simulink library "Hydraulic_Actuator_Lib"  (R2019b)
settings: Solver=ode45  StartTime=0.0  StopTime=10.0  RelTol=1e-3  EnableMultiTasking=on
undefined symbols (not defined in the file): WT_Params
libraries: fl_lib x15, sh_lib x9, nesl_utility x9, fl_ps_legacy_lib x4
Description:
  | Copyright 2009-2017 The MathWorks, Inc. MathWorks, Inc.
settings Model: Creator=smiller  LastModifiedBy=bhisma
settings DataIOCC: LimitDataPoints=on  SaveFormat=Array  SignalLoggingSaveFormat=ModelDataLogs  ReturnWorkspaceOutputs=off
settings OptimizationCC: ExpressionDepthLimit=2147483647  LifeSpan=inf
settings DebuggingCC: UnderspecifiedInitializationDetection=Classic  MergeDetectMultiDrivingBlocksExec=none  SolverPrmCheckMsg=warning  FcnCallInpInsideContextMsg=warning  AllowSymbolicDim=off  StateNameClashWarn=warning  SFUnexpectedBacktrackingDiag=warning  SFNoUnconditionalDefaultTransitionDiag=warning  SFExecutionAtInitializationDiag=none  ArithmeticOperatorsInVariantConditions=warning
settings HardwareCC: ProdBitPerPointer=32  ProdBitPerSizeT=32  ProdBitPerPtrDiffT=32  ProdLargestAtomicFloat=None  ProdIntDivRoundTo=Undefined  ProdEndianess=Unspecified  ProdWordSize=32  ProdHWDeviceType=32-bit Generic
settings ModelReferenceCC: PropagateSignalLabelsOutOfModel=off
settings SFSimCC: SimUseLocalCustomCode=off  CustomCodeUndefinedFunction=UseInterfaceOnly
settings RTWCC: RTWUseLocalCustomCode=off
settings CodeAppCC: StateflowObjectComments=on
settings GRTTargetCC: TargetLangStandard=C89/C90 (ANSI)  GeneratePreprocessorConditionals=Disable all  CombineOutputUpdateFcns=off  GRTInterface=on
settings ConfigComp: CovMetricSettings=dw  CovHtmlReporting=on  CovSaveCumulativeToWorkspaceVar=on  CovSaveSingleToWorkspaceVar=on  CovExternalEMLEnable=off  CovSFcnEnable=off

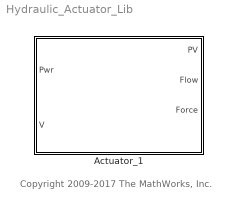
== system Hydraulic_Actuator_Lib ==
  note: Copyright 2009-2017 The MathWorks, Inc.
  Actuator_1 : Subsystem
      mask Display: image(imread('Pitch_Hydraulic_Actuator_IMAGE.jpg'));

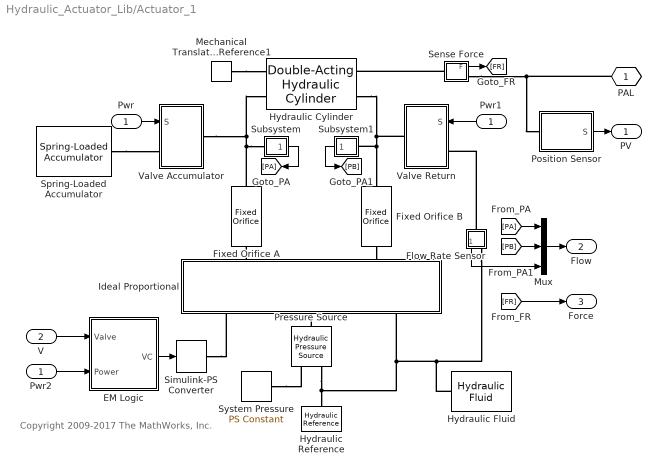
== system Hydraulic_Actuator_Lib/Actuator_1 ==
  note: Copyright 2009-2017 The MathWorks, Inc.
  Pwr : Inport
  V : Inport  Port=2
  EM Logic : Subsystem
  Fixed Orifice A : sh_lib/Orifices/Fixed Orifice  area=WT_Params.Pitch_Actuator.orifice_area m^2  C_d=0.7  lam_spec=2  B_lam=0.999  Re_cr=12  q_specify=off  q_priority=High  q=1 m^3/s  q_nominal_specify=off  q_nominal_unit=m^3/s  q_nominal_value=1  p_specify=off  p_priority=High  p=0 Pa  p_nominal_specify=off  p_nominal_unit=Pa  p_nominal_value=1
      settings: SourceProductName=Simscape Fluids  SourceProductBaseCode=SH  InternalSimscapePortConfiguration="{\"Bottom\":[],\"Left\":[{\"id\":\"A\",\"label\":\"A\",\"type\":\"foundation.hydraulic.hydraulic\"}],\"Right\":[{\"id\":\"B\",\"label\":\"B\",\"type\":\"foundation.hydraulic.hydraulic\"}],\"Top\":[]}"
  Fixed Orifice B : sh_lib/Orifices/Fixed Orifice  area=WT_Params.Pitch_Actuator.orifice_area m^2  C_d=0.7  lam_spec=2  B_lam=0.999  Re_cr=12  q_specify=off  q_priority=High  q=1 m^3/s  q_nominal_specify=off  q_nominal_unit=m^3/s  q_nominal_value=1  p_specify=off  p_priority=High  p=0 Pa  p_nominal_specify=off  p_nominal_unit=Pa  p_nominal_value=1
      settings: SourceProductName=Simscape Fluids  SourceProductBaseCode=SH  InternalSimscapePortConfiguration="{\"Bottom\":[],\"Left\":[{\"id\":\"A\",\"label\":\"A\",\"type\":\"foundation.hydraulic.hydraulic\"}],\"Right\":[{\"id\":\"B\",\"label\":\"B\",\"type\":\"foundation.hydraulic.hydraulic\"}],\"Top\":[]}"
  Flow Rate Sensor : Subsystem
      mask Display: disp('F')
  Hydraulic Reference : fl_lib/Hydraulic/Hydraulic Elements/Hydraulic Reference
      settings: SourceProductName=Simscape
  Hydraulic Cylinder : sh_lib/Hydraulic Cylinders/Double-Acting Hydraulic Cylinder  area_A=WT_Params.Pitch_Actuator.Cylinder.piston_area m^2  area_B=WT_Params.Pitch_Actuator.Cylinder.piston_area m^2  stroke=WT_Params.Pitch_Actuator.Cylinder.stroke m  init_pos=WT_Params.Pitch_Actuator.Cylinder.initial_disp_from_a m  dead_vol_A=1e-04 m^3  dead_vol_B=1e-04 m^3  init_pressure_A=0 Pa  init_pressure_B=0 Pa  k_sh=1.4  stiff=WT_Params.Pitch_Actuator.Cylinder.contact_stiffness N/m  D=WT_Params.Pitch_Actuator.Cylinder.contact_damping N/(m/s)  hardstop_model=3  transition=0.1 mm  or=2
      settings: SourceProductName=Simscape Fluids  SourceProductBaseCode=SH  InternalSimscapePortConfiguration="{\"Bottom\":[],\"Left\":[{\"id\":\"C\",\"label\":\"C\",\"type\":\"foundation.mechanical.translational.translational\"},{\"id\":\"A\",\"label\":\"A\",\"type\":\"foundation.hydraulic.hydraulic\"}],\"Right\":[{\"id\":\"R\",\"label\":\"R\",\"type\":\"foundation.mechanical.translational.translational\"},{\"id\":\"B\",\"label\":\"B\",\"type\":\"foundation.hydraulic.hydraulic\"}],\"Top\":[]}"
  Hydraulic Fluid : sh_lib/Hydraulic Utilities/Hydraulic Fluid  DataSource=1  SelFluid=1  SysTemp=60  TrapAir=0.005  ViscDerFactor=1  range_error=2
      settings: SourceProductName=Simscape Fluids
  Ideal Proportional : Subsystem
      mask Display:
      | plot([198.418507352471;198.418507352471], [5.66910021007061;25.5109509453177])
      | plot([189.914857037365;206.922157667577], [25.5109509453177;25.5109509453177])
      | plot([240.936758928001;240.936758928001], [5.66910021007061;25.5109509453177])
      | plot([232.433108612895;249.440409243107], [25.5109509453177;25.5109509453177])
      | plot([240.936758928001;240.936758928001], [76.5328528359532;56.6910021007061])
      | plot([232.433108612895;249.440409243107], [56.6910021007061;56.6910021007061])
      | plot([198.418507352471;198.418507352471], [76.5328528359532;56.6910021007061])
      | plot([189.914857037365;206.922157667577], [56.6910021007061;56.6910021007061])
      | plot([99.2092536762357;99.2092536762357], [76.5328528359532;5.66910021007061])
      | plot([141.727505251765;141.727505251765], [76.5328528359532;5.66910021007061])
      | plot([170.073006302118;170.073006302118], [76.5328528359532;5.66910021007061])
      | plot([269.282259978354;269.282259978354], [76.5328528359532;5.66910021007061])
      | patch([99.2092536762357;93.5401534661651;104.878353886306;99.2092536762357], [76.5328528359532;53.8564519956708;53.8564519956708;76.5328528359532],[0 0 0])
      | plot([99.2092536762357;93.5401534661651;104.878353886306;99.2092536762357], [76.5328528359532;53.8564519956708;53.8564519956708;76.5328528359532])
      | patch([141.727505251765;136.058405041695;147.396605461836;141.727505251765], [5.66910021007061;28.3455010503531;28.3455010503531;5.66910021007061],[0 0 0])
      | plot([141.727505251765;136.058405041695;147.396605461836;141.727505251765], [5.66910021007061;28.3455010503531;28.3455010503531;5.66910021007061])
      | plot([297.627761028707;340.146012604237], [5.66910021007061;76.5328528359532])
      | plot([297.627761028707;340.146012604237], [76.5328528359532;5.66910021007061])
      | plot([70.8637526258826;368.49151365459;368.49151365459;70.8637526258826;70.8637526258826], [76.5328528359532;76.5328528359532;5.66910021007061;5.66910021007061;76.5328528359532])
      | patch([297.627761028707;303.296861238778;311.800511553884;297.627761028707], [5.66910021007061;25.5109509453177;19.8418507352471;5.66910021007061],[0 0 0])
      | plot([297.627761028707;303.296861238778;311.800511553884;297.627761028707], [5.66910021007061;25.5109509453177;19.8418507352471;5.66910021007061])
      | patch([297.627761028707;303.296861238778;311.800511553884;297.627761028707], [76.5328528359532;56.6910021007061;62.3601023107767;76.5328528359532],[0 0 0])
      | plot([297.627761028707;303.296861238778;311.800511553884;297.627761028707], [76.5328528359532;56.6910021007061;62.3601023107767;76.5328528359532])
      | plot([62.3601023107767;374.16061386466], [82.2019530460238;82.2019530460238])
      | plot([65.194652415812;376.995163969696], [0;0])
      | plot([70.8637526258826;0;0;70.8637526258826;70.8637526258826], [53.8564519956708;53.8564519956708;25.5109509453177;25.5109509453177;53.8564519956708]-25.5109509453177+5.66910021007061)
      | plot([70.8637526258826;0;0;70.8637526258826;70.8637526258826]+368.49151365459, [53.8564519956708;53.8564519956708;25.5109509453177;25.5109509453177;53.8564519956708]-25.5109509453177+5.66910021007061)
      | plot([15 25], [5.66910021007061 35])
      | plot([25 15]+405, [5.66910021007061 35])
      | plot([42.5 40]+5,[70 58]);
      | plot([45 50]+2.5,[70 45]);
      | plot([45 50]+7.5,[45 70]);
      | plot([45 50]+12.5,[70 45]);
      | plot([45 50]+17.5,[45 70]);
      | plot([40 42.5]+27.5,[70 58]);
      | plot([42.5 40]+5+324,[70 58]);
      | plot([45 50]+2.5+324,[70 45]);
      | plot([45 50]+7.5+324,[45 70]);
      | plot([45 50]+12.5+324,[70 45]);
      | plot([45 50]+17.5+324,[45 70]);
      | plot([40 42.5]+27.5+324,[70 58]);
      | ;color('red');
      | port_label('LConn', 1,'A')
      | port_label('LConn', 2,'B')
      | port_label('RConn', 1,'S')
      | port_label('RConn', 2,'P')
      | port_label('RConn', 3,'T')
  Mechanical Translational Reference1 : fl_lib/Mechanical/Translational Elements/Mechanical Translational Reference  Tag=Factory Generic
  Mux : Mux  Inputs=3
  Position Sensor : Subsystem
      mask Display:
      | plot([25.5109509453177;56.6910021007061;70.8637526258826;96.3747035712004;127.554754726589;155.900255776942;184.245756827295;212.591257877648;235.26765871793;252.274959348142;283.455010503531], [155.900255776942;155.900255776942;110.547454096377;198.418507352471;113.382004201412;198.418507352471;116.216554306448;198.418507352471;113.382004201412;155.900255776942;155.900255776942])
      | plot([155.900255776942;155.900255776942], [266.447709873319;198.418507352471])
      | patch([155.900255776942;170.073006302118;141.727505251765;155.900255776942], [198.418507352471;226.764008402824;226.764008402824;198.418507352471], [0;0;0])
      | plot([155.900255776942;170.073006302118;141.727505251765;155.900255776942], [198.418507352471;226.764008402824;226.764008402824;198.418507352471])
      | ;
      | color('red');
      | port_label('LConn', 1,'R')
      | port_label('output', 1,'P')
  Pressure Source : fl_lib/Hydraulic/Hydraulic Sources/Hydraulic Pressure Source
      settings: SourceProductName=Simscape  SourceProductBaseCode=SS  InternalSimscapePortConfiguration="{\"Bottom\":[],\"Left\":[{\"id\":\"P\",\"label\":\"P\",\"type\":\"foundation.hydraulic.hydraulic\"}],\"Right\":[{\"id\":\"S\",\"label\":\"S\",\"type\":\"input\"},{\"id\":\"T\",\"label\":\"T\",\"type\":\"foundation.hydraulic.hydraulic\"}],\"Top\":[]}"
  Pwr1 : InportShadow
  Pwr2 : InportShadow
  Sense Force : Subsystem
      mask Display: disp('F');
  Simulink-PS Converter : nesl_utility/Simulink-PS Converter  PhysicalDomain=network_engine_domain  SubClassName=ps_input  LeftPortType=input  RightPortType=output  PseudoPeriodic=off  Frequencies=[]  NoiseDistribution=none  NoiseParameters=[]  Unit=1  AffineConversion=off  FilteringAndDerivatives=zero  SimscapeFilterOrder=1  InputFilterTimeConstant=.001  UdotUserProvided=0
  Spring-Loaded Accumulator : sh_lib/Accumulators/Spring-Loaded Accumulator  capacity=WT_Params.Pitch_Actuator.Accumulator.capacity m^3  pr_preload=WT_Params.Pitch_Actuator.Accumulator.preload_pressure Pa  pr_max=WT_Params.Pitch_Actuator.Accumulator.maximum_pressure Pa  stiff_coeff=0 Pa/m^3  penetr_coeff=1e15 s*Pa/m^6  flow_rate_specify=off  flow_rate_priority=None  flow_rate=0.005 m^3/s  flow_rate_nominal_specify=off  flow_rate_nominal_unit=m^3/s  flow_rate_nominal_value=1  fluid_volume_specify=on  fluid_volume_priority=High  fluid_volume=WT_Params.Pitch_Actuator.Accumulator.initial_volume m^3  fluid_volume_nominal_specify=off  fluid_volume_nominal_unit=m^3  fluid_volume_nominal_value=1  fluid_pressure_specify=off  fluid_pressure_priority=None  fluid_pressure=1.01325e+5 Pa  fluid_pressure_nominal_specify=off  fluid_pressure_nominal_unit=Pa  fluid_pressure_nominal_value=1
      settings: SourceProductName=Simscape Fluids  SourceProductBaseCode=SH  InternalSimscapePortConfiguration="{\"Bottom\":[],\"Left\":[],\"Right\":[{\"id\":\"A\",\"label\":\"A\",\"type\":\"foundation.hydraulic.hydraulic\"}],\"Top\":[]}"
  Subsystem : Subsystem
      mask Display: disp('P')
  Subsystem1 : Subsystem
      mask Display: disp('P')
  System Pressure : fl_lib/Physical Signals/Sources/PS Constant  constant=WT_Params.Pitch_Actuator.hydraulic_pressure
  Valve Accumulator : Subsystem
      mask Display:
      | plot([73.6983027309179;124.720204621553], [181.41120672226;181.41120672226])
      | plot([76.2808928266168;277.78591029346], [385.498814284801;385.498814284801])
      | plot([77.0997628569603;276.967040263116], [283.455010503531;283.455010503531])
      | plot([73.6983027309179;276.967040263116;276.967040263116;73.6983027309179;73.6983027309179], [487.542618066072;487.542618066072;79.3674029409885;79.3674029409885;487.542618066072])
      | plot([277.78591029346;226.764008402824], [181.41120672226;181.285226717591])
      | plot([226.764008402824;226.764008402824], [205.28441760689;157.286035828292])
      | patch([206.35524764657;206.35524764657;280.368500389159;206.35524764657], [400.805384851992;370.192243717611;385.498814284801;400.805384851992], [0;0;0])
      | plot([206.35524764657;206.35524764657;280.368500389159;206.35524764657], [400.805384851992;370.192243717611;385.498814284801;400.805384851992])
      | plot([124.720204621553;124.720204621553], [204.906477592885;156.971085816622])
      | plot([0;351.484213024378;351.484213024378;0;0], [566.910021007061;566.910021007061;0;0;566.910021007061])
      | ;
      | color('red');
      | port_label('input', 1,'S');
      | port_label('lconn', 1,'A');
      | port_label('rconn', 1,'B');
  Valve Return : Subsystem
      mask Display:
      | plot([73.6983027309179;124.720204621553], [181.41120672226;181.41120672226])
      | plot([76.2808928266168;277.78591029346], [385.498814284801;385.498814284801])
      | plot([77.0997628569603;276.967040263116], [283.455010503531;283.455010503531])
      | plot([73.6983027309179;276.967040263116;276.967040263116;73.6983027309179;73.6983027309179], [487.542618066072;487.542618066072;79.3674029409885;79.3674029409885;487.542618066072])
      | plot([277.78591029346;226.764008402824], [181.41120672226;181.285226717591])
      | plot([226.764008402824;226.764008402824], [205.28441760689;157.286035828292])
      | patch([206.35524764657;206.35524764657;280.368500389159;206.35524764657], [400.805384851992;370.192243717611;385.498814284801;400.805384851992], [0;0;0])
      | plot([206.35524764657;206.35524764657;280.368500389159;206.35524764657], [400.805384851992;370.192243717611;385.498814284801;400.805384851992])
      | plot([124.720204621553;124.720204621553], [204.906477592885;156.971085816622])
      | plot([0;351.484213024378;351.484213024378;0;0], [566.910021007061;566.910021007061;0;0;566.910021007061])
      | ;
      | color('red');
      | port_label('input', 1,'S');
      | port_label('lconn', 1,'A');
      | port_label('rconn', 1,'B');
  PAL : PMIOPort  Tag=PMCPort  Side=Right
  PV : Outport
  Flow : Outport  Port=2
  Force : Outport  Port=3
  wires:
  Pwr2/1 -> EM Logic/2(Power)
  EM Logic/1(VC) -> Simulink-PS Converter/1
  [PB] -> Mux/2
  [PA] -> Mux/1
  Flow Rate Sensor/1(Flow) -> Mux/3
  Subsystem1/1(P) -> [PB]
  Subsystem/1(P) -> [PA]
  V/1 -> EM Logic/1(Valve)
  Pwr1/1 -> Valve Return/1(S)
  Pwr/1 -> Valve Accumulator/1(S)
  Position Sensor/1(S) -> PV/1
  Mux/1 -> Flow/1
  Sense Force/1(F) -> [FR]
  [FR] -> Force/1
  connections:
  Flow Rate Sensor/LConn1 -- Valve Return/LConn1
  Sense Force/RConn1 -- PAL/RConn1 -- Position Sensor/LConn1
  Spring-Loaded Accumulator/RConn1 -- Valve Accumulator/LConn1
  Mechanical Translational Reference1/LConn1 -- Hydraulic Cylinder/LConn1
  Subsystem/LConn1 -- Fixed Orifice A/RConn1 -- Valve Accumulator/RConn1 -- Hydraulic Cylinder/LConn2
  Subsystem1/LConn1 -- Valve Return/RConn1 -- Hydraulic Cylinder/RConn2 -- Fixed Orifice B/RConn1
  Ideal Proportional/LConn1 -- Fixed Orifice A/LConn1
  Fixed Orifice B/LConn1 -- Ideal Proportional/LConn2
  Ideal Proportional/RConn3 -- Hydraulic Reference/LConn1 -- Pressure Source/RConn2 -- Hydraulic Fluid/RConn1 -- Flow Rate Sensor/RConn1
  Simulink-PS Converter/RConn1 -- Ideal Proportional/RConn1
  Pressure Source/LConn1 -- Ideal Proportional/RConn2
  System Pressure/RConn1 -- Pressure Source/RConn1
  Sense Force/LConn1 -- Hydraulic Cylinder/RConn1

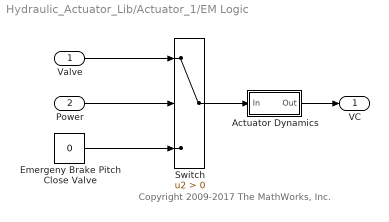
== system Hydraulic_Actuator_Lib/Actuator_1/EM Logic ==
  note: Copyright 2009-2017 The MathWorks, Inc.
  Valve : Inport
  Power : Inport  Port=2
  Actuator Dynamics : Subsystem  mask(First-order lag supporting vector signals){b=WT_Params.Pitch_Actuator.hydraulic_actuator_time_constant, x_initial=0}
      mask prompts: b "Filter time constant"; x_initial "Initial output"
      mask help: Models a lag of the form 1/(b*s+1) where s is the Laplace operator.
  Emergeny Brake Pitch Close Valve : Constant  Value=0
  Switch : Switch  Criteria=u2 > Threshold
  VC : Outport
  wires:
  Switch/1 -> Actuator Dynamics/1(In)
  Emergeny Brake Pitch Close Valve/1 -> Switch/3
  Power/1 -> Switch/2
  Valve/1 -> Switch/1
  Actuator Dynamics/1(Out) -> VC/1

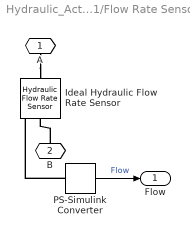
== system Hydraulic_Actuator_Lib/Actuator_1/Flow Rate Sensor ==
  Ideal Hydraulic Flow Rate Sensor : fl_lib/Hydraulic/Hydraulic Sensors/Hydraulic Flow Rate Sensor
      settings: SourceProductName=Simscape
  PS-Simulink Converter : nesl_utility/PS-Simulink Converter  PhysicalDomain=network_engine_domain  SubClassName=ps_output  LeftPortType=input  RightPortType=output  PseudoPeriodic=off  Frequencies=[]  Unit=1  AffineConversion=off
  A : PMIOPort  Side=Left
  B : PMIOPort  Port=2  Side=Right
  Flow : Outport
  wires:
  PS-Simulink Converter/1 -> Flow/1  "Flow"
  connections:
  B/RConn1 -- Ideal Hydraulic Flow Rate Sensor/RConn2
  A/RConn1 -- Ideal Hydraulic Flow Rate Sensor/LConn1
  PS-Simulink Converter/LConn1 -- Ideal Hydraulic Flow Rate Sensor/RConn1

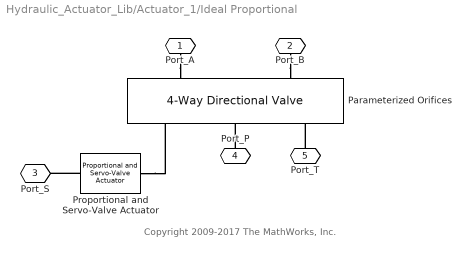
== system Hydraulic_Actuator_Lib/Actuator_1/Ideal Proportional ==
  note: Copyright 2009-2017 The MathWorks, Inc.
  Parameterized Orifices : sh_lib/Valves/Directional Valves/4-Way Directional Valve  area_spec=1  x_0_P_A=WT_Params.Pitch_Actuator.Valve.initial_opening_pa m  x_0_P_B=WT_Params.Pitch_Actuator.Valve.initial_opening_pb m  x_0_A_T=WT_Params.Pitch_Actuator.Valve.initial_opening_at m  x_0_B_T=WT_Params.Pitch_Actuator.Valve.initial_opening_bt m  mdl_type_identical=1  mdl_type_different=1  opening_max=WT_Params.Pitch_Actuator.Valve.max_opening m  area_max=WT_Params.Pitch_Actuator.Valve.max_area m^2  opening_max_P_A=0.005 m  area_max_P_A=0.5e-4 m^2  opening_max_P_B=0.005 m  area_max_P_B=0.5e-4 m^2  opening_max_A_T=0.005 m  area_max_A_T=0.5e-4 m^2  opening_max_B_T=0.005 m  area_max_B_T=0.5e-4 m^2  opening_area_tab="[  -0.002 0 0.002 0.005 0.015 ] m"  area_tab="[  1e-09 2.0352e-07 4.0736e-05 0.00011438 0.00034356 ] m^2"  opening_flow_rate_tab="[  -0.002 0 0.002 0.005 0.015 ] m"  pressure_tab="[  -1e+07 -5e+06 -2e+06 2e+06 5e+06 1e+07 ] Pa"  flow_rate_tab="[  -1e-07 -7.0711e-08 -4.4721e-08 4.4721e-08 7.0711e-08 1e-07 ; -2.0352e-05 -1.4391e-05 -9.1017e-06 9.1017e-06 1.4391e-05 2.0352e-05 ; -0.0040736 -0.0028805 -0.0018218 0.0018218 0.0028805 0.0040736 ; -0.011438 -0.0080879 -0.0051152 0.0051152 0.0080879 0.011438 ; -0.034356 -0.024293 -0.015364 0.015364 0.024293 0.034356 ; ] m^3/s"  opening_area_tab_P_A=[-0.002, 0.0, 0.002, 0.005, 0.015] m  area_tab_P_A=[1.0e-9, 2.0352e-7, 4.0736e-5, 0.00011438, 0.00034356] m^2  opening_flow_rate_tab_P_A=[-0.002, 0.0, 0.002, 0.005, 0.015] m  pressure_tab_P_A=[-10000000.0, -5000000.0, -2000000.0, 2000000.0, 5000000.0, 10000000.0] Pa  flow_rate_tab_P_A=[-1.0e-7, -7.0711e-8, -4.4721e-8, 4.4721e-8, 7.0711e-8, 1.0e-7; -2.0352e-5, -1.4391e-5, -9.1017e-6, 9.1017e-6, 1.4391e-5, 2.0352e-5; -0.0040736, -0.0028805, -0.0018218, 0.0018218, 0.0028805, 0.0040736; -0.011438, -0.0080879, -0.0051152, 0.0051152, 0.0080879, 0.011438; -0.034356, -0.024293, -0.015364, 0.015364, 0.024293, 0.034356] m^3/s  opening_area_tab_P_B=[-0.002, 0.0, 0.002, 0.005, 0.015] m  area_tab_P_B=[1.0e-9, 2.0352e-7, 4.0736e-5, 0.00011438, 0.00034356] m^2  opening_flow_rate_tab_P_B=[-0.002, 0.0, 0.002, 0.005, 0.015] m  pressure_tab_P_B=[-10000000.0, -5000000.0, -2000000.0, 2000000.0, 5000000.0, 10000000.0] Pa  flow_rate_tab_P_B=[-1.0e-7, -7.0711e-8, -4.4721e-8, 4.4721e-8, 7.0711e-8, 1.0e-7; -2.0352e-5, -1.4391e-5, -9.1017e-6, 9.1017e-6, 1.4391e-5, 2.0352e-5; -0.0040736, -0.0028805, -0.0018218, 0.0018218, 0.0028805, 0.0040736; -0.011438, -0.0080879, -0.0051152, 0.0051152, 0.0080879, 0.011438; -0.034356, -0.024293, -0.015364, 0.015364, 0.024293, 0.034356] m^3/s  opening_area_tab_A_T=[-0.002, 0.0, 0.002, 0.005, 0.015] m  area_tab_A_T=[1.0e-9, 2.0352e-7, 4.0736e-5, 0.00011438, 0.00034356] m^2  opening_flow_rate_tab_A_T=[-0.002, 0.0, 0.002, 0.005, 0.015] m  pressure_tab_A_T=[-10000000.0, -5000000.0, -2000000.0, 2000000.0, 5000000.0, 10000000.0] Pa  flow_rate_tab_A_T=[-1.0e-7, -7.0711e-8, -4.4721e-8, 4.4721e-8, 7.0711e-8, 1.0e-7; -2.0352e-5, -1.4391e-5, -9.1017e-6, 9.1017e-6, 1.4391e-5, 2.0352e-5; -0.0040736, -0.0028805, -0.0018218, 0.0018218, 0.0028805, 0.0040736; -0.011438, -0.0080879, -0.0051152, 0.0051152, 0.0080879, 0.011438; -0.034356, -0.024293, -0.015364, 0.015364, 0.024293, 0.034356] m^3/s  opening_area_tab_B_T=[-0.002, 0.0, 0.002, 0.005, 0.015] m  area_tab_B_T=[1.0e-9, 2.0352e-7, 4.0736e-5, 0.00011438, 0.00034356] m^2  opening_flow_rate_tab_B_T=[-0.002, 0.0, 0.002, 0.005, 0.015] m  pressure_tab_B_T=[-10000000.0, -5000000.0, -2000000.0, 2000000.0, 5000000.0, 10000000.0] Pa  flow_rate_tab_B_T=[-1.0e-7, -7.0711e-8, -4.4721e-8, 4.4721e-8, 7.0711e-8, 1.0e-7; -2.0352e-5, -1.4391e-5, -9.1017e-6, 9.1017e-6, 1.4391e-5, 2.0352e-5; -0.0040736, -0.0028805, -0.0018218, 0.0018218, 0.0028805, 0.0040736; -0.011438, -0.0080879, -0.0051152, 0.0051152, 0.0080879, 0.011438; -0.034356, -0.024293, -0.015364, 0.015364, 0.024293, 0.034356] m^3/s  interp_method_identical=1  interp_method_different=1  extrap_method_identical=1  extrap_method_different=1  A_leak=WT_Params.Pitch_Actuator.Valve.leakage_area m^2  C_d=0.7  lam_spec=2  B_lam=0.999  Re_cr=12
      settings: SourceProductName=Simscape Fluids  SourceProductBaseCode=SH  InternalSimscapePortConfiguration="{\"Bottom\":[],\"Left\":[{\"id\":\"A\",\"label\":\"A\",\"type\":\"foundation.hydraulic.hydraulic\"},{\"id\":\"B\",\"label\":\"B\",\"type\":\"foundation.hydraulic.hydraulic\"}],\"Right\":[{\"id\":\"S\",\"label\":\"S\",\"type\":\"input\"},{\"id\":\"P\",\"label\":\"P\",\"type\":\"foundation.hydraulic.hydraulic\"},{\"id\":\"T\",\"label\":\"T\",\"type\":\"foundation.hydraulic.hydraulic\"}],\"Top\":[]}"
  Proportional and Servo-Valve Actuator : sh_lib/Valves/Valve Actuators/Proportional and Servo-Valve Actuator  gain=WT_Params.Pitch_Actuator.Servo.gain  time_constant=WT_Params.Pitch_Actuator.Servo.time_constant s  saturation=WT_Params.Pitch_Actuator.Servo.saturation
      settings: SourceProductName=Simscape Fluids  SourceProductBaseCode=SH  InternalSimscapePortConfiguration="{\"Bottom\":[],\"Left\":[{\"id\":\"I\",\"label\":\"\",\"type\":\"input\"}],\"Right\":[{\"id\":\"O\",\"label\":\"\",\"type\":\"output\"}],\"Top\":[]}"
  Port_A : PMIOPort  Side=Left
  Port_B : PMIOPort  Port=2  Side=Left
  Port_S : PMIOPort  Port=3  Side=Right
  Port_P : PMIOPort  Port=4  Side=Right
  Port_T : PMIOPort  Port=5  Side=Right
  connections:
  Port_A/RConn1 -- Parameterized Orifices/LConn1
  Port_B/RConn1 -- Parameterized Orifices/LConn2
  Proportional and Servo-Valve Actuator/RConn1 -- Parameterized Orifices/RConn1
  Port_P/RConn1 -- Parameterized Orifices/RConn2
  Port_T/RConn1 -- Parameterized Orifices/RConn3
  Proportional and Servo-Valve Actuator/LConn1 -- Port_S/RConn1

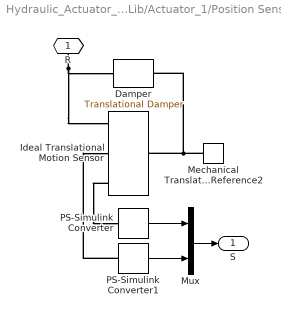
== system Hydraulic_Actuator_Lib/Actuator_1/Position Sensor ==
  Damper : fl_lib/Mechanical/Translational Elements/Translational Damper  D=WT_Params.Pitch_Actuator.Cylinder.damping N/(m/s)  v_specify=off  v_priority=High  v=0 m/s  v_nominal_specify=off  v_nominal_unit=m/s  v_nominal_value=1  f_specify=off  f_priority=High  f=0 N  f_nominal_specify=off  f_nominal_unit=N  f_nominal_value=1
  Ideal Translational Motion Sensor : fl_lib/Mechanical/Mechanical Sensors/Ideal Translational Motion Sensor  offset=WT_Params.Pitch_Actuator.Sensor.initial_position m
  Mechanical Translational Reference2 : fl_lib/Mechanical/Translational Elements/Mechanical Translational Reference  Tag=Factory Generic
  Mux : Mux  Inputs=2
  PS-Simulink Converter : nesl_utility/PS-Simulink Converter  PhysicalDomain=network_engine_domain  SubClassName=ps_output  LeftPortType=input  RightPortType=output  PseudoPeriodic=off  Frequencies=[]  Unit=1  AffineConversion=off
  PS-Simulink Converter1 : nesl_utility/PS-Simulink Converter  PhysicalDomain=network_engine_domain  SubClassName=ps_output  LeftPortType=input  RightPortType=output  PseudoPeriodic=off  Frequencies=[]  Unit=1  AffineConversion=off
  R : PMIOPort  Side=Left
  S : Outport
  wires:
  PS-Simulink Converter1/1 -> Mux/2
  Mux/1 -> S/1
  PS-Simulink Converter/1 -> Mux/1
  connections:
  PS-Simulink Converter1/LConn1 -- Ideal Translational Motion Sensor/RConn2
  Ideal Translational Motion Sensor/RConn3 -- PS-Simulink Converter/LConn1
  Mechanical Translational Reference2/LConn1 -- Ideal Translational Motion Sensor/LConn1 -- Damper/RConn1
  R/RConn1 -- Damper/LConn1 -- Ideal Translational Motion Sensor/RConn1

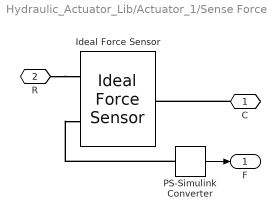
== system Hydraulic_Actuator_Lib/Actuator_1/Sense Force ==
  Ideal Force Sensor : fl_lib/Mechanical/Mechanical Sensors/Ideal Force Sensor
  PS-Simulink Converter : nesl_utility/PS-Simulink Converter  PhysicalDomain=network_engine_domain  SubClassName=ps_output  LeftPortType=input  RightPortType=output  PseudoPeriodic=off  Frequencies=[]  Unit=1  AffineConversion=off
  C : PMIOPort  Side=Right
  R : PMIOPort  Port=2  Side=Left
  F : Outport
  wires:
  PS-Simulink Converter/1 -> F/1
  connections:
  PS-Simulink Converter/LConn1 -- Ideal Force Sensor/RConn2
  C/RConn1 -- Ideal Force Sensor/LConn1
  R/RConn1 -- Ideal Force Sensor/RConn1

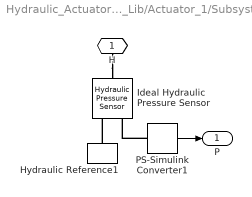
== system Hydraulic_Actuator_Lib/Actuator_1/Subsystem ==
  Hydraulic Reference1 : fl_lib/Hydraulic/Hydraulic Elements/Hydraulic Reference
      settings: SourceProductName=Simscape
  Ideal Hydraulic Pressure Sensor : fl_lib/Hydraulic/Hydraulic Sensors/Hydraulic Pressure Sensor
      settings: SourceProductName=Simscape
  PS-Simulink Converter1 : nesl_utility/PS-Simulink Converter  PhysicalDomain=network_engine_domain  SubClassName=ps_output  LeftPortType=input  RightPortType=output  PseudoPeriodic=off  Frequencies=[]  Unit=1  AffineConversion=off
  H : PMIOPort  Side=Left
  P : Outport
  wires:
  PS-Simulink Converter1/1 -> P/1
  connections:
  H/RConn1 -- Ideal Hydraulic Pressure Sensor/LConn1
  PS-Simulink Converter1/LConn1 -- Ideal Hydraulic Pressure Sensor/RConn2
  Hydraulic Reference1/LConn1 -- Ideal Hydraulic Pressure Sensor/RConn1

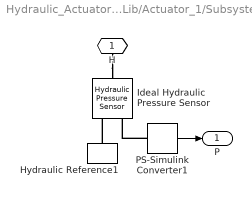
== system Hydraulic_Actuator_Lib/Actuator_1/Subsystem1 ==
  Hydraulic Reference1 : fl_lib/Hydraulic/Hydraulic Elements/Hydraulic Reference
      settings: SourceProductName=Simscape
  Ideal Hydraulic Pressure Sensor : fl_lib/Hydraulic/Hydraulic Sensors/Hydraulic Pressure Sensor
      settings: SourceProductName=Simscape
  PS-Simulink Converter1 : nesl_utility/PS-Simulink Converter  PhysicalDomain=network_engine_domain  SubClassName=ps_output  LeftPortType=input  RightPortType=output  PseudoPeriodic=off  Frequencies=[]  Unit=1  AffineConversion=off
  H : PMIOPort  Side=Left
  P : Outport
  wires:
  PS-Simulink Converter1/1 -> P/1
  connections:
  Hydraulic Reference1/LConn1 -- Ideal Hydraulic Pressure Sensor/RConn1
  PS-Simulink Converter1/LConn1 -- Ideal Hydraulic Pressure Sensor/RConn2
  H/RConn1 -- Ideal Hydraulic Pressure Sensor/LConn1

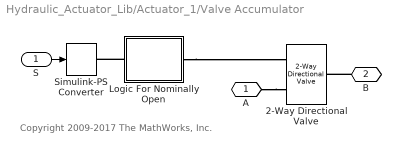
== system Hydraulic_Actuator_Lib/Actuator_1/Valve Accumulator ==
  note: Copyright 2009-2017 The MathWorks, Inc.
  S : Inport
  2-Way Directional Valve : sh_lib/Valves/Directional Valves/2-Way Directional Valve  mdl_type=1  area_max=WT_Params.Pitch_Actuator.Emergency_Pitch_Valve.max_area m^2  opening_max=0.005 m  opening_tab="[  -0.002 0 0.002 0.005 0.015 ] m"  area_tab="[  1e-09 2.0352e-07 4.0736e-05 0.00011438 0.00034356 ] m^2"  pressure_tab="[  -1e+07 -5e+06 -2e+06 2e+06 5e+06 1e+07 ] Pa"  flow_rate_tab="[  -1e-07 -7.0711e-08 -4.4721e-08 4.4721e-08 7.0711e-08 1e-07 ; -2.0352e-05 -1.4391e-05 -9.1017e-06 9.1017e-06 1.4391e-05 2.0352e-05 ; -0.0040736 -0.0028805 -0.0018218 0.0018218 0.0028805 0.0040736 ; -0.011438 -0.0080879 -0.0051152 0.0051152 0.0080879 0.011438 ; -0.034356 -0.024293 -0.015364 0.015364 0.024293 0.034356 ; ] m^3/s"  interp_method=1  extrap_method=1  C_d=0.7  x_0=0 m  A_leak=1e-12 m^2  lam_spec=2  B_lam=0.999  Re_cr=12
      settings: SourceProductName=Simscape Fluids  SourceProductBaseCode=SH  InternalSimscapePortConfiguration="{\"Bottom\":[],\"Left\":[{\"id\":\"S\",\"label\":\"S\",\"type\":\"input\"},{\"id\":\"A\",\"label\":\"A\",\"type\":\"foundation.hydraulic.hydraulic\"}],\"Right\":[{\"id\":\"B\",\"label\":\"B\",\"type\":\"foundation.hydraulic.hydraulic\"}],\"Top\":[]}"
  Logic For Nominally Open : Subsystem
  Simulink-PS Converter : nesl_utility/Simulink-PS Converter  PhysicalDomain=network_engine_domain  SubClassName=ps_input  LeftPortType=input  RightPortType=output  PseudoPeriodic=off  Frequencies=[]  NoiseDistribution=none  NoiseParameters=[]  Unit=1  AffineConversion=off  FilteringAndDerivatives=zero  SimscapeFilterOrder=1  InputFilterTimeConstant=.001  UdotUserProvided=0
  A : PMIOPort  Side=Left
  B : PMIOPort  Port=2  Side=Right
  wires:
  S/1 -> Simulink-PS Converter/1
  connections:
  Logic For Nominally Open/RConn1 -- 2-Way Directional Valve/LConn1
  B/RConn1 -- 2-Way Directional Valve/RConn1
  A/RConn1 -- 2-Way Directional Valve/LConn2
  Logic For Nominally Open/LConn1 -- Simulink-PS Converter/RConn1

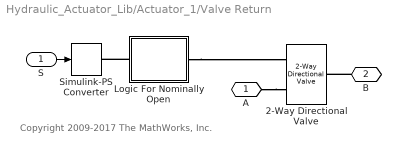
== system Hydraulic_Actuator_Lib/Actuator_1/Valve Return ==
  note: Copyright 2009-2017 The MathWorks, Inc.
  S : Inport
  2-Way Directional Valve : sh_lib/Valves/Directional Valves/2-Way Directional Valve  mdl_type=1  area_max=WT_Params.Pitch_Actuator.Emergency_Pitch_Valve.max_area m^2  opening_max=0.005 m  opening_tab="[  -0.002 0 0.002 0.005 0.015 ] m"  area_tab="[  1e-09 2.0352e-07 4.0736e-05 0.00011438 0.00034356 ] m^2"  pressure_tab="[  -1e+07 -5e+06 -2e+06 2e+06 5e+06 1e+07 ] Pa"  flow_rate_tab="[  -1e-07 -7.0711e-08 -4.4721e-08 4.4721e-08 7.0711e-08 1e-07 ; -2.0352e-05 -1.4391e-05 -9.1017e-06 9.1017e-06 1.4391e-05 2.0352e-05 ; -0.0040736 -0.0028805 -0.0018218 0.0018218 0.0028805 0.0040736 ; -0.011438 -0.0080879 -0.0051152 0.0051152 0.0080879 0.011438 ; -0.034356 -0.024293 -0.015364 0.015364 0.024293 0.034356 ; ] m^3/s"  interp_method=1  extrap_method=1  C_d=0.7  x_0=0 m  A_leak=1e-12 m^2  lam_spec=2  B_lam=0.999  Re_cr=12
      settings: SourceProductName=Simscape Fluids  SourceProductBaseCode=SH  InternalSimscapePortConfiguration="{\"Bottom\":[],\"Left\":[{\"id\":\"S\",\"label\":\"S\",\"type\":\"input\"},{\"id\":\"A\",\"label\":\"A\",\"type\":\"foundation.hydraulic.hydraulic\"}],\"Right\":[{\"id\":\"B\",\"label\":\"B\",\"type\":\"foundation.hydraulic.hydraulic\"}],\"Top\":[]}"
  Logic For Nominally Open : Subsystem
  Simulink-PS Converter : nesl_utility/Simulink-PS Converter  PhysicalDomain=network_engine_domain  SubClassName=ps_input  LeftPortType=input  RightPortType=output  PseudoPeriodic=off  Frequencies=[]  NoiseDistribution=none  NoiseParameters=[]  Unit=1  AffineConversion=off  FilteringAndDerivatives=zero  SimscapeFilterOrder=1  InputFilterTimeConstant=.001  UdotUserProvided=0
  A : PMIOPort  Side=Left
  B : PMIOPort  Port=2  Side=Right
  wires:
  S/1 -> Simulink-PS Converter/1
  connections:
  Logic For Nominally Open/LConn1 -- Simulink-PS Converter/RConn1
  A/RConn1 -- 2-Way Directional Valve/LConn2
  B/RConn1 -- 2-Way Directional Valve/RConn1
  Logic For Nominally Open/RConn1 -- 2-Way Directional Valve/LConn1

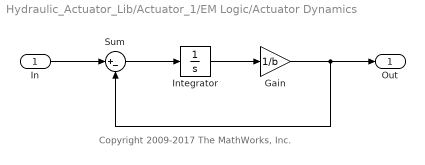
== system Hydraulic_Actuator_Lib/Actuator_1/EM Logic/Actuator Dynamics ==
  note: Copyright 2009-2017 The MathWorks, Inc.
  In : Inport
  Gain : Gain  Gain=1/b
  Integrator : Integrator  InitialCondition=x_initial
  Sum : Sum  Inputs=|+-  SaturateOnIntegerOverflow=on  InputSameDT=on  OutDataTypeStr=Inherit: Same as first input
  Out : Outport
  wires:
  Gain/1 -> Out/1, Sum/2
  Integrator/1 -> Gain/1
  In/1 -> Sum/1
  Sum/1 -> Integrator/1

== system Hydraulic_Actuator_Lib/Actuator_1/Valve Accumulator/Logic For Nominally Open ==
  PS Gain : fl_ps_legacy_lib/Legacy Physical Signals/Functions/PS Gain  gain=-1
      settings: SourceProductName=Simscape
  PS Subtract : fl_ps_legacy_lib/Legacy Physical Signals/Functions/PS Subtract
      settings: SourceProductName=Simscape  SourceProductBaseCode=SS
  Voltage_Open : fl_lib/Physical Signals/Sources/PS Constant  constant=24
  S : PMIOPort  Side=Left
  VA : PMIOPort  Port=2  Side=Right
  connections:
  VA/RConn1 -- PS Gain/RConn1
  S/RConn1 -- PS Subtract/LConn1
  PS Subtract/RConn1 -- PS Gain/LConn1
  PS Subtract/LConn2 -- Voltage_Open/RConn1

== system Hydraulic_Actuator_Lib/Actuator_1/Valve Return/Logic For Nominally Open ==
  PS Gain : fl_ps_legacy_lib/Legacy Physical Signals/Functions/PS Gain  gain=-1
      settings: SourceProductName=Simscape
  PS Subtract : fl_ps_legacy_lib/Legacy Physical Signals/Functions/PS Subtract
      settings: SourceProductName=Simscape  SourceProductBaseCode=SS
  Voltage_Open : fl_lib/Physical Signals/Sources/PS Constant  constant=24
  S : PMIOPort  Side=Left
  VA : PMIOPort  Port=2  Side=Right
  connections:
  PS Subtract/LConn2 -- Voltage_Open/RConn1
  PS Subtract/RConn1 -- PS Gain/LConn1
  S/RConn1 -- PS Subtract/LConn1
  VA/RConn1 -- PS Gain/RConn1
